simulink model "lot_vol"  (R2024b)
settings: Solver=VariableStepAuto  StartTime=0.0  StopTime=10.0  RelTol=1e-3
settings Model: Creator=foxjustfox  LastModifiedBy=foxjustfox

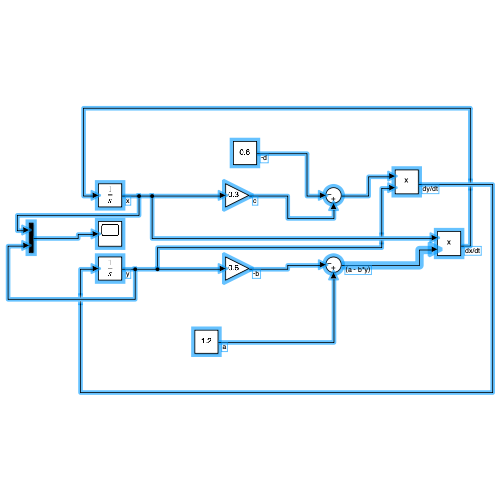
[thumbnail: Simulink's stored preview of the top-level diagram]
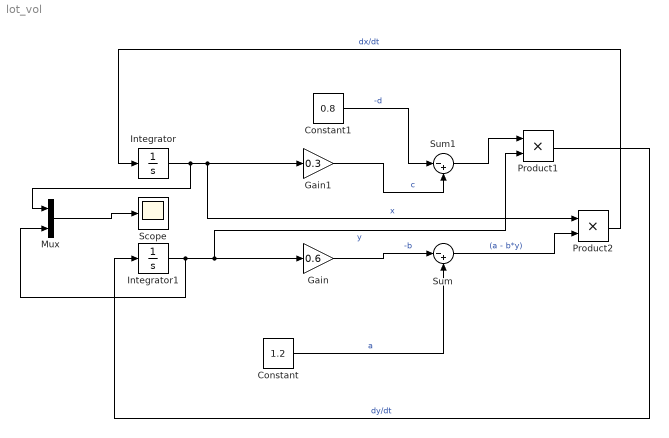
== system lot_vol ==
  Constant : Constant  Value=1.2
  Constant1 : Constant  Value=0.8
  Gain : Gain  Gain=0.6
  Gain1 : Gain  Gain=0.3
  Integrator : Integrator  InitialCondition=2
  Integrator1 : Integrator  InitialCondition=1
  Mux : Mux  Inputs=2
  Product1 : Product
  Product2 : Product
  Scope : Scope
  Sum : Sum  Inputs=|-+
  Sum1 : Sum  Inputs=|-+
  wires:
  Sum1/1 -> Product1/1
  Integrator1/1 -> Mux/2, Product1/2, Gain/1  "y"
  Integrator/1 -> Gain1/1, Product2/1, Mux/1  "x"
  Product2/1 -> Integrator/1  "dx/dt"
  Constant1/1 -> Sum1/1  "-d"
  Constant/1 -> Sum/2  "a"
  Gain/1 -> Sum/1  "-b"
  Gain1/1 -> Sum1/2  "c"
  Mux/1 -> Scope/1
  Product1/1 -> Integrator1/1  "dy/dt"
  Sum/1 -> Product2/2  "(a - b*y)"
